simulink model "matlabfunc"  (R2015a)
settings: Solver=ode45  StartTime=0.0  StopTime=20  RelTol=1e-3
values from neighbouring files (symbols this model uses):
  x0 = [0.2; 0.4]    [set_params_matlabfunc.m]
undefined symbols (not defined in the file or in its folder): parSys
libraries: cstblocks x1
settings Model: Creator=am  LastModifiedBy=zp
settings OptimizationCC: ExpressionDepthLimit=2147483647
settings DebuggingCC: UnderspecifiedInitializationDetection=Classic  MergeDetectMultiDrivingBlocksExec=none  SolverPrmCheckMsg=warning  StateNameClashWarn=warning

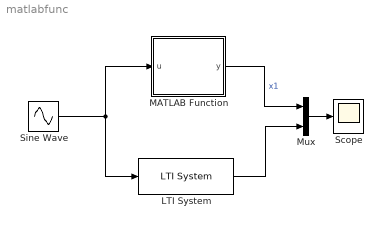
== system matlabfunc ==
  LTI System : cstblocks/LTI System  sys=sysd  IC=x0
  MATLAB Function : MATLAB Function  TreatAsAtomicUnit=on
  Mux : Mux  Inputs=2
  Scope : Scope
      settings: TimeRange=10  YMin=-0.1  YMax=0.6
  Sine Wave : Sin  SampleTime=0
  wires:
  Sine Wave/1 -> LTI System/1, MATLAB Function/1(u)
  MATLAB Function/1(y) -> Mux/1  "x1"
  LTI System/1 -> Mux/2
  Mux/1 -> Scope/1

== matlab function matlabfunc/MATLAB Function ==
  settings: updateMethod=DISCRETE  sampleTime=Ta
  data: u input; x0 parameter; y output; parSys parameter
function y = fcn(u, x0, parSys)
%#codegen
% ------------------------------------------------------------------------
% Initialisierung der persistenten Variablen
% ------------------------------------------------------------------------

% Zustand
persistent x;
if(isempty(x))
    x = x0;
end

% ------------------------------------------------------------------------
% Programm
% ------------------------------------------------------------------------

% Loesen des zeitdiskreten Systems
y = parSys.C*x+parSys.D*u;
x = parSys.Phi*x+parSys.Gamma*u;
